simulink model "Controller"  (R2022b)
settings: Solver=VariableStepAuto  StartTime=t(1)  StopTime=t(end)  RelTol=1e-3
values from neighbouring files (symbols this model uses):
  K_P = 1    [Analysis.m]
  KC = 0.05    [Analysis.m]
  T_d = 30    [Analysis.m]
  T_i = 0.001    [Analysis.m]
settings Model: Creator=debber  LastModifiedBy=debber
settings DataIOCC: LoadExternalInput=on  SaveFormat=Array  OutputSaveName=y

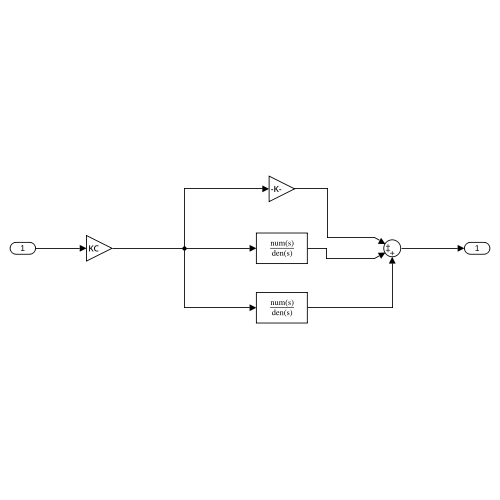
[thumbnail: Simulink's stored preview of the top-level diagram]
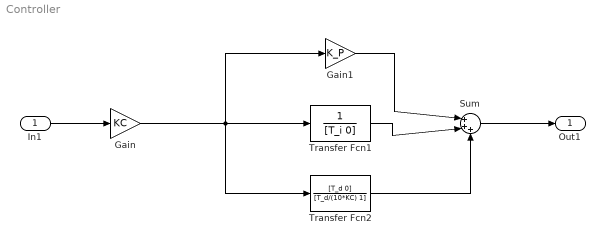
== system Controller ==
  In1 : Inport
  Gain : Gain  Gain=KC
  Gain1 : Gain  Gain=K_P
  Sum : Sum  Inputs=|+++
  Transfer Fcn1 : TransferFcn  Denominator=[T_i 0]
  Transfer Fcn2 : TransferFcn  Numerator=[T_d 0]  Denominator=[T_d/(10*KC) 1]
  Out1 : Outport
  wires:
  In1/1 -> Gain/1
  Gain/1 -> Gain1/1, Transfer Fcn2/1, Transfer Fcn1/1
  Gain1/1 -> Sum/1
  Transfer Fcn1/1 -> Sum/2
  Transfer Fcn2/1 -> Sum/3
  Sum/1 -> Out1/1
